simulink model "High_Striker_Simulink_Matlab"  (R2013a)
settings: Solver=ode3  SolverMode=SingleTasking  StartTime=0.0  StopTime=10.0  RelTol=1e-3
libraries: arduinolib x3, simulink x1
settings Model: ExtModeTrigDuration=2  Creator=cgupta  LastModifiedBy=ankit
settings OptimizationCC: OptimizeModelRefInitCode=on  LifeSpan=1
settings DebuggingCC: SolverPrmCheckMsg=none  StrictBusMsg=Warning
settings HardwareCC: ProdBitPerInt=16  ProdBitPerPointer=8  ProdIntDivRoundTo=Zero  ProdEndianess=LittleEndian  ProdWordSize=8  ProdHWDeviceType=Atmel->AVR
settings RTWCC: SystemTargetFile=realtime.tlc  GenerateMakefile=off  TemplateMakefile=realtime.tmf  Description=Run on Target Hardware  RTWVerbose=off  ProcessScript=realtime_make_rtw_hook
settings STFCustomTargetCC: TargetLibSuffix=.a  GenerateSampleERTMain=on  ERTCustomFileBanners=on  SupportNonInlinedSFcns=off  SupportVariableSizeSignals=on  MATLABClassNameForMDSCustomization=Simulink.SoftwareTarget.ERTCustomization  SystemTargetFile=realtime.tlc
settings ERTTargetCC: ParMdlRefBuildCompliant=off  CompOptLevelCompliant=off  ConcurrentExecutionCompliant=off  CombineOutputUpdateFcns=off  ERTFirstTimeCompliant=off  SupportContinuousTime=on  SupportVariableSizeSignals=on  ModelStepFunctionPrototypeControlCompliant=off  CPPClassGenCompliant=off  ExtModeTransport=3  ExtModeMexFile=ext_serial_win32_comm  ExtModeMexArgs=0 1 9600  ERTSrcFileBannerTemplate=realtime_code_template.cgt  ERTHdrFileBannerTemplate=realtime_code_template.cgt  ERTDataSrcFileTemplate=realtime_code_template.cgt  ERTDataHdrFileTemplate=realtime_code_template.cgt  ERTCustomFileTemplate=realtime_file_process.tlc

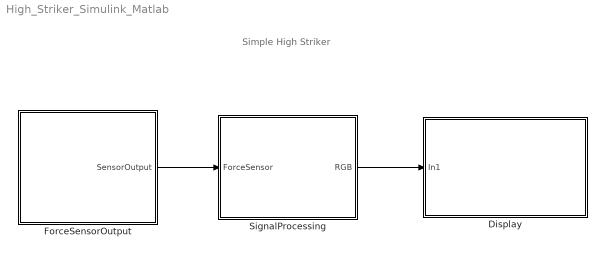
== system High_Striker_Simulink_Matlab ==
  note: Simple High Striker
  Display : Subsystem
  ForceSensorOutput : Subsystem
  SignalProcessing : Subsystem
  wires:
  ForceSensorOutput/1(SensorOutput) -> SignalProcessing/1(ForceSensor)
  SignalProcessing/1(RGB) -> Display/1(In1)

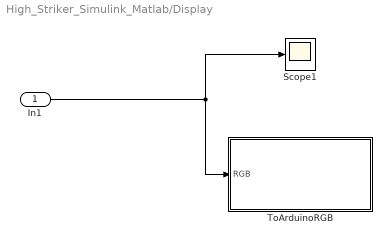
== system High_Striker_Simulink_Matlab/Display ==
  In1 : Inport
  Scope1 : Scope
      settings: TimeRange=600  YMin=-50  YMax=300
  ToArduinoRGB : Subsystem
  wires:
  In1/1 -> Scope1/1, ToArduinoRGB/1(RGB)

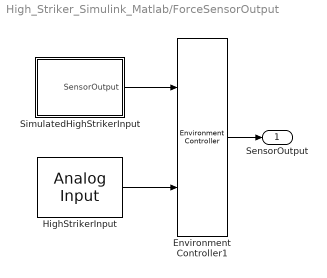
== system High_Striker_Simulink_Matlab/ForceSensorOutput ==
  Environment Controller1 : simulink/Signal Routing/Environment Controller
  HighStrikerInput : arduinolib/Analog Input  pinNumber=0  sampleTime=0.2
  SimulatedHighStrikerInput : Subsystem
  SensorOutput : Outport
  wires:
  HighStrikerInput/1 -> Environment Controller1/2
  Environment Controller1/1 -> SensorOutput/1
  SimulatedHighStrikerInput/1(SensorOutput) -> Environment Controller1/1

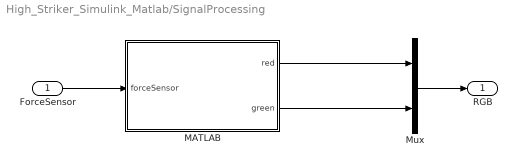
== system High_Striker_Simulink_Matlab/SignalProcessing ==
  ForceSensor : Inport
  MATLAB : MATLAB Function  TreatAsAtomicUnit=on
  Mux : Mux  Inputs=2
  RGB : Outport
  wires:
  Mux/1 -> RGB/1
  ForceSensor/1 -> MATLAB/1(forceSensor)
  MATLAB/1(red) -> Mux/1
  MATLAB/2(green) -> Mux/2

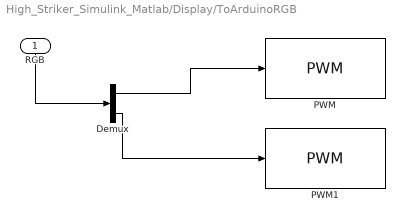
== system High_Striker_Simulink_Matlab/Display/ToArduinoRGB ==
  RGB : Inport
  Demux : Demux  Outputs=2
  PWM : arduinolib/PWM  pinNumber=11
  PWM1 : arduinolib/PWM  pinNumber=10
  wires:
  Demux/2 -> PWM1/1
  Demux/1 -> PWM/1
  RGB/1 -> Demux/1

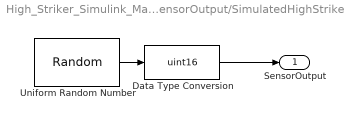
== system High_Striker_Simulink_Matlab/ForceSensorOutput/SimulatedHighStrikerInput ==
  Data Type Conversion : DataTypeConversion  OutDataTypeStr=uint16  SaturateOnIntegerOverflow=on
  Uniform Random Number : UniformRandomNumber  Minimum=0  Maximum=1023  SampleTime=0.1
  SensorOutput : Outport
  wires:
  Uniform Random Number/1 -> Data Type Conversion/1
  Data Type Conversion/1 -> SensorOutput/1

== matlab function High_Striker_Simulink_Matlab/SignalProcessing/MATLAB ==
  data: forceSensor input; red output; green output
function [red, green] = FSR2RGB(forceSensor)
%#codegen

% Red : As the FSR increases red goes to zero
% Green increases as FSR increases
red = int8(255 - forceSensor/3); % Some bias on red
green = int8(forceSensor/4);
